simulink model "Modelo_obs_y_acelerometro_escalon"  (R2020a)
settings: Solver=ode15s  StartTime=0.0  StopTime=5  FixedStep=0.001  MaxStep=1/fs  RelTol=1e-3
undefined symbols (not defined in the file): A, A_reduc, Amp, B, B_reduc, ba, Bdlol, C_reduc, Cc, D, f0, fs, I_max, K_motor_virtual, ksi, ksia, L, Li, Lobs, obs_i_den, obs_i_num, obs_x2_den, obs_x2_num, R, R_control, v0, w_acc, x0, zita_acc, ZOH
libraries: simulink x1, dspstat3 x1
settings Model: Creator=Noxi-PC  LastModifiedBy=Noxi-PC

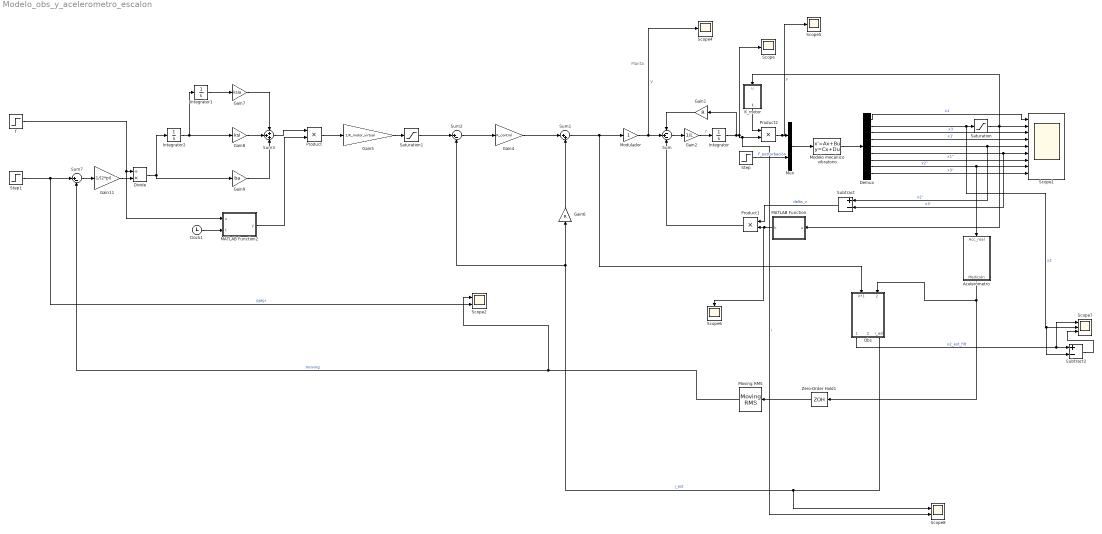
== system Modelo_obs_y_acelerometro_escalon ==
  note: Planta
  Acelerómetro : Subsystem
  Clock1 : Clock
  Demux : Demux  Outputs=9
  Divide : Product  Inputs=/*
  Gain1 : Gain  Gain=R
  Gain11 : Gain  Gain=1/(2*pi)
  Gain2 : Gain  Gain=1/L
  Gain4 : Gain  Gain=R_control
  Gain5 : Gain  Gain=1/K_motor_virtual
  Gain6 : Gain  Gain=R
  Gain7 : Gain  Gain=ksia
  Gain8 : Gain  Gain=ksi
  Gain9 : Gain  Gain=ba
  Integrator : Integrator
  Integrator1 : Integrator
  Integrator2 : Integrator
  K_motor : MATLAB Function  TreatAsAtomicUnit=on
  MATLAB Function : MATLAB Function  TreatAsAtomicUnit=on
  MATLAB Function2 : MATLAB Function  TreatAsAtomicUnit=on
  Modelo mecánico vibratorio : StateSpace  A=A  B=B  C=Cc  D=D  InitialCondition=[x0,v0]
  Modulador : Gain
  Moving RMS : dspstat3/Moving RMS  Method=Sliding window  ForgettingFactorPort=off  SpecifyWindowLength=on  WindowLength=Ventana  ForgettingFactor=0.99  SimulateUsing=Code generation
      settings: SourceProductBaseCode=DS
  Mux : Mux  Inputs=2
  Obs : Subsystem
  Product : Product
  Product1 : Product
  Product2 : Product
  Saturation : Saturate  UpperLimit=12.7e-3  LowerLimit=-12.7e-3
  Saturation1 : Saturate  UpperLimit=I_max  LowerLimit=-I_max
  Scope{,4..6} (4 alike) : Scope
  Scope1 : Scope  NumInputPorts=9
  Scope2 : Scope  NumInputPorts=2
  Scope7 : Scope  NumInputPorts=3
  Scope8 : Scope  NumInputPorts=2
  Step : Step  Time=3  After=0  SampleTime=0
  Step1 : Step  After=Amp/sqrt(2)  SampleTime=0
  Subtract : Sum  Inputs=+-
  Subtract2 : Sum  Inputs=+-
  Sum : Sum  Inputs=-+-
  Sum1 : Sum  Inputs=|++
  Sum2 : Sum  Inputs=|+-
  Sum3 : Sum  Inputs=+++
  Sum7 : Sum  Inputs=|+-
  Zero-Order Hold1 : ZeroOrderHold  SampleTime=ZOH
  f : Step  Time=0  After=f0  SampleTime=0
  wires:
  Modelo mecánico vibratorio/1 -> Demux/1
  Demux/1 -> Scope1/1  "x1"
  Demux/2 -> Subtract2/2, Scope7/2, Saturation/1  "x2"
  Demux/3 -> Scope1/3  "x3"
  Demux/4 -> Scope1/4  "x1'"
  Demux/5 -> Scope1/5, Subtract/1  "x2'"
  Demux/6 -> Scope1/6, Subtract/2  "x3'"
  Demux/7 -> Scope1/7  "x1''"
  Demux/8 -> Acelerómetro/1(Acc_real), Scope1/8  "x2''"
  Demux/9 -> Scope1/9  "x3''"
  Mux/1 -> Modelo mecánico vibratorio/1
  Sum/1 -> Gain2/1
  Integrator/1 -> Scope8/2, Product2/2, Scope/1, Gain1/1  "i"
  Gain1/1 -> Sum/1
  Gain2/1 -> Integrator/1  "i'"
  Step/1 -> Mux/2  "F_perturbación"
  Product1/1 -> Sum/3
  Subtract/1 -> Product1/1  "delta_v"
  Modulador/1 -> Scope4/1, Sum/2  "V"
  Sum2/1 -> Gain4/1
  Gain5/1 -> Saturation1/1
  Gain4/1 -> Sum1/1
  Gain8/1 -> Sum3/2
  Gain7/1 -> Sum3/1
  Gain9/1 -> Sum3/3
  Integrator1/1 -> Gain7/1
  Integrator2/1 -> Integrator1/1, Gain8/1
  Acelerómetro/1(Medición) -> Zero-Order Hold1/1, Obs/2(acc_medida1)
  Zero-Order Hold1/1 -> Moving RMS/1
  Step1/1 -> Scope2/2, Sum7/1  "RMS*"
  Moving RMS/1 -> Scope2/1, Sum7/2  "moving"
  Sum7/1 -> Gain11/1
  Sum3/1 -> Product/1
  Saturation/1 -> K_motor/1(u), MATLAB Function/1(u), Scope1/2
  Product2/1 -> Scope5/1, Mux/1  "F"
  K_motor/1(k) -> Product2/1
  MATLAB Function/1(k) -> Scope6/1, Product1/2
  Sum1/1 -> Obs/1(V*1), Modulador/1
  Divide/1 -> Gain9/1, Integrator2/1
  Gain11/1 -> Divide/2
  Product/1 -> Gain5/1
  Saturation1/1 -> Sum2/1
  f/1 -> MATLAB Function2/1(u), Divide/1
  MATLAB Function2/1(y) -> Product/2
  Clock1/1 -> MATLAB Function2/2(t)
  Gain6/1 -> Sum1/2
  Obs/3(i_est) -> Scope8/1, Gain6/1, Sum2/2  "i_est"
  Subtract2/1 -> Scope7/3
  Obs/1(x2_est) -> Scope7/1, Subtract2/1  "x2_est_filt"

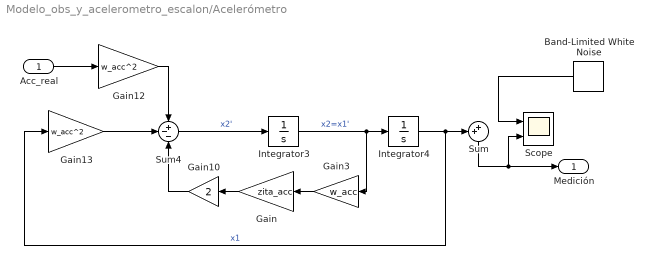
== system Modelo_obs_y_acelerometro_escalon/Acelerómetro ==
  Acc_real : Inport
  Band-Limited White Noise : simulink/Sources/Band-Limited White Noise  Cov=NoisePower  Ts=1/fs  seed=[23341]
  Gain : Gain  Gain=zita_acc
  Gain10 : Gain  Gain=2
  Gain12 : Gain  Gain=w_acc^2
  Gain13 : Gain  Gain=w_acc^2
  Gain3 : Gain  Gain=w_acc
  Integrator3 : Integrator
  Integrator4 : Integrator
  Scope : Scope  NumInputPorts=2
  Sum : Sum  Inputs=++|
  Sum4 : Sum  Inputs=+--
  Medición : Outport
  wires:
  Gain/1 -> Gain10/1
  Integrator4/1 -> Gain13/1, Sum/1  "x1"
  Acc_real/1 -> Gain12/1
  Gain12/1 -> Sum4/1
  Sum4/1 -> Integrator3/1  "x2'"
  Gain3/1 -> Gain/1
  Integrator3/1 -> Integrator4/1, Gain3/1  "x2=x1'"
  Gain13/1 -> Sum4/2
  Gain10/1 -> Sum4/3
  Sum/1 -> Scope/2, Medición/1
  Band-Limited White Noise/1 -> Scope/1

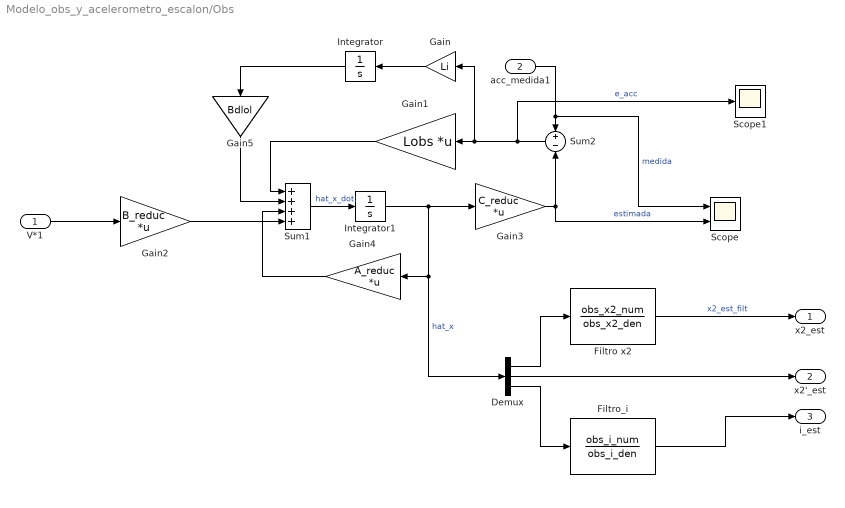
== system Modelo_obs_y_acelerometro_escalon/Obs ==
  V*1 : Inport
  acc_medida1 : Inport  Port=2
  Demux : Demux  Outputs=3
  Filtro x2 : TransferFcn  Numerator=obs_x2_num  Denominator=obs_x2_den
  Filtro_i : TransferFcn  Numerator=obs_i_num  Denominator=obs_i_den
  Gain : Gain  Gain=Li
  Gain1 : Gain  Gain=Lobs  Multiplication=Matrix(K*u)
  Gain2 : Gain  Gain=B_reduc  Multiplication=Matrix(K*u)
  Gain3 : Gain  Gain=C_reduc  Multiplication=Matrix(K*u)
  Gain4 : Gain  Gain=A_reduc  Multiplication=Matrix(K*u)
  Gain5 : Gain  Gain=Bdlol
  Integrator : Integrator
  Integrator1 : Integrator
  Scope : Scope  NumInputPorts=2
  Scope1 : Scope
  Sum1 : Sum  Inputs=++++
  Sum2 : Sum  Inputs=+|-
  x2_est : Outport
  x2'_est : Outport  Port=2
  i_est : Outport  Port=3
  wires:
  Gain1/1 -> Sum1/1
  Gain4/1 -> Sum1/3
  V*1/1 -> Gain2/1
  Sum2/1 -> Scope1/1, Gain/1, Gain1/1  "e_acc"
  Integrator1/1 -> Demux/1, Gain4/1, Gain3/1  "hat_x"
  Sum1/1 -> Integrator1/1  "hat_x_dot"
  acc_medida1/1 -> Scope/1, Sum2/1  "medida"
  Gain3/1 -> Sum2/2, Scope/2  "estimada"
  Gain/1 -> Integrator/1
  Integrator/1 -> Gain5/1
  Gain5/1 -> Sum1/2
  Gain2/1 -> Sum1/4
  Demux/1 -> Filtro x2/1
  Filtro x2/1 -> x2_est/1  "x2_est_filt"
  Demux/2 -> x2'_est/1
  Demux/3 -> Filtro_i/1
  Filtro_i/1 -> i_est/1

== matlab function Modelo_obs_y_acelerometro_escalon/MATLAB Function ==
  data: u input; k output
function k= fcn(u)
coefs = [1883883250149.81,121220914.941173,-604988778.285297,-369001.905871325,-43371.4523559472,-47.4444922489166,51.4222931299995];

k = coefs(1)*u^6+coefs(2)*u^5+coefs(3)*u^4+coefs(4)*u^3+coefs(5)*u^2+coefs(6)*u^1+coefs(7);

== matlab function Modelo_obs_y_acelerometro_escalon/MATLAB Function2 ==
  data: u input; y output; t input
function y = fcn(u,t)

y = sin(2*pi*u*t);

== matlab function Modelo_obs_y_acelerometro_escalon/K_motor ==
  data: u input; k output
function k = fcn(u)
coefs = [1.88388325014986e-06,1.21220914940963e-07,-0.000604988778285308,-0.000369001905871298,-0.0433714523559467,-0.0474444922489168,51.4222931299995];

k = coefs(1)*u^6+coefs(2)*u^5+coefs(3)*u^4+coefs(4)*u^3+coefs(5)*u^2+coefs(6)*u^1+coefs(7);
